simulink model "gm_parallel_lht_vnl"  (R2019b)
settings: Solver=FixedStepDiscrete  StartTime=0.0  StopTime=inf  RelTol=1e-3
undefined symbols (not defined in the file or in its folder): bt, height, nTheta, width
libraries: hdlsllib x199, simulink x27, hdlmdlgenlib x7, dspsrcs4 x1
(part 4 of 19)

== system gm_parallel_lht_vnl/Parallel LHT/Parallel LHT Accumulator/Accumulator with Switches/Accumulator_instance125 ==
  mode : Inport  OutDataTypeStr=boolean  PortDimensions=1  SampleTime=6.66666666666667e-09
  address : Inport  Port=2  OutDataTypeStr=fixdt(0, 9, 0)  PortDimensions=1  SampleTime=6.66666666666667e-09
  edge : Inport  Port=3  OutDataTypeStr=boolean  PortDimensions=1  SampleTime=6.66666666666667e-09
  AND : Logic  IconShape=distinctive  AllPortsSameDT=off  OutDataTypeStr=boolean
  Add : Sum  OutDataTypeStr=fixdt(0, ceil(log2(maxRho*2)), 0)
  Block RAM : Subsystem
  Delay{,1..3} (4 alike) : Delay  DelayLength=1
  Multiport Switch : MultiPortSwitch  DataPortOrder=Zero-based contiguous  Inputs=2  zeroidx=on
  Multiport Switch1 : MultiPortSwitch  DataPortOrder=Zero-based contiguous  Inputs=2  zeroidx=on
  Relational Operator : RelationalOperator  Operator===  OutDataTypeStr=boolean  RndMeth=Simplest
  Vote : Constant  OutDataTypeStr=fixdt(0,1,0)  SampleTime=-1
  Zero : Constant  OutDataTypeStr=fixdt(0,1,0)  SampleTime=-1
  hps : Outport
  wires:
  Zero/1 -> Multiport Switch/2
  Vote/1 -> Add/1
  Relational Operator/1 -> AND/2
  Delay2/1 -> Multiport Switch1/1
  Delay1/1 -> AND/1, Block RAM/3(wr_en)
  Delay/1 -> Relational Operator/1, Block RAM/2(wr_addr)
  Block RAM/1(rd_data) -> hps/1, Multiport Switch1/2
  AND/1 -> Delay2/1
  mode/1 -> Multiport Switch/1
  address/1 -> Relational Operator/2, Delay/1, Block RAM/4(rd_addr)
  edge/1 -> Delay1/1
  Multiport Switch/1 -> Block RAM/1(wr_data)
  Delay3/1 -> Multiport Switch1/3
  Multiport Switch1/1 -> Add/2
  Add/1 -> Multiport Switch/3, Delay3/1

== system gm_parallel_lht_vnl/Parallel LHT/Parallel LHT Accumulator/Accumulator with Switches/Accumulator_instance126 ==
  mode : Inport  OutDataTypeStr=boolean  PortDimensions=1  SampleTime=6.66666666666667e-09
  address : Inport  Port=2  OutDataTypeStr=fixdt(0, 9, 0)  PortDimensions=1  SampleTime=6.66666666666667e-09
  edge : Inport  Port=3  OutDataTypeStr=boolean  PortDimensions=1  SampleTime=6.66666666666667e-09
  AND : Logic  IconShape=distinctive  AllPortsSameDT=off  OutDataTypeStr=boolean
  Add : Sum  OutDataTypeStr=fixdt(0, ceil(log2(maxRho*2)), 0)
  Block RAM : Subsystem
  Delay{,1..3} (4 alike) : Delay  DelayLength=1
  Multiport Switch : MultiPortSwitch  DataPortOrder=Zero-based contiguous  Inputs=2  zeroidx=on
  Multiport Switch1 : MultiPortSwitch  DataPortOrder=Zero-based contiguous  Inputs=2  zeroidx=on
  Relational Operator : RelationalOperator  Operator===  OutDataTypeStr=boolean  RndMeth=Simplest
  Vote : Constant  OutDataTypeStr=fixdt(0,1,0)  SampleTime=-1
  Zero : Constant  OutDataTypeStr=fixdt(0,1,0)  SampleTime=-1
  hps : Outport
  wires:
  Zero/1 -> Multiport Switch/2
  Vote/1 -> Add/1
  Relational Operator/1 -> AND/2
  Delay2/1 -> Multiport Switch1/1
  Delay1/1 -> AND/1, Block RAM/3(wr_en)
  Delay/1 -> Relational Operator/1, Block RAM/2(wr_addr)
  Block RAM/1(rd_data) -> hps/1, Multiport Switch1/2
  AND/1 -> Delay2/1
  mode/1 -> Multiport Switch/1
  address/1 -> Relational Operator/2, Delay/1, Block RAM/4(rd_addr)
  edge/1 -> Delay1/1
  Multiport Switch/1 -> Block RAM/1(wr_data)
  Delay3/1 -> Multiport Switch1/3
  Multiport Switch1/1 -> Add/2
  Add/1 -> Multiport Switch/3, Delay3/1

== system gm_parallel_lht_vnl/Parallel LHT/Parallel LHT Accumulator/Accumulator with Switches/Accumulator_instance127 ==
  mode : Inport  OutDataTypeStr=boolean  PortDimensions=1  SampleTime=6.66666666666667e-09
  address : Inport  Port=2  OutDataTypeStr=fixdt(0, 9, 0)  PortDimensions=1  SampleTime=6.66666666666667e-09
  edge : Inport  Port=3  OutDataTypeStr=boolean  PortDimensions=1  SampleTime=6.66666666666667e-09
  AND : Logic  IconShape=distinctive  AllPortsSameDT=off  OutDataTypeStr=boolean
  Add : Sum  OutDataTypeStr=fixdt(0, ceil(log2(maxRho*2)), 0)
  Block RAM : Subsystem
  Delay{,1..3} (4 alike) : Delay  DelayLength=1
  Multiport Switch : MultiPortSwitch  DataPortOrder=Zero-based contiguous  Inputs=2  zeroidx=on
  Multiport Switch1 : MultiPortSwitch  DataPortOrder=Zero-based contiguous  Inputs=2  zeroidx=on
  Relational Operator : RelationalOperator  Operator===  OutDataTypeStr=boolean  RndMeth=Simplest
  Vote : Constant  OutDataTypeStr=fixdt(0,1,0)  SampleTime=-1
  Zero : Constant  OutDataTypeStr=fixdt(0,1,0)  SampleTime=-1
  hps : Outport
  wires:
  Zero/1 -> Multiport Switch/2
  Vote/1 -> Add/1
  Relational Operator/1 -> AND/2
  Delay2/1 -> Multiport Switch1/1
  Delay1/1 -> AND/1, Block RAM/3(wr_en)
  Delay/1 -> Relational Operator/1, Block RAM/2(wr_addr)
  Block RAM/1(rd_data) -> hps/1, Multiport Switch1/2
  AND/1 -> Delay2/1
  mode/1 -> Multiport Switch/1
  address/1 -> Relational Operator/2, Delay/1, Block RAM/4(rd_addr)
  edge/1 -> Delay1/1
  Multiport Switch/1 -> Block RAM/1(wr_data)
  Delay3/1 -> Multiport Switch1/3
  Multiport Switch1/1 -> Add/2
  Add/1 -> Multiport Switch/3, Delay3/1

== system gm_parallel_lht_vnl/Parallel LHT/Parallel LHT Accumulator/Accumulator with Switches/Accumulator_instance128 ==
  mode : Inport  OutDataTypeStr=boolean  PortDimensions=1  SampleTime=6.66666666666667e-09
  address : Inport  Port=2  OutDataTypeStr=fixdt(0, 9, 0)  PortDimensions=1  SampleTime=6.66666666666667e-09
  edge : Inport  Port=3  OutDataTypeStr=boolean  PortDimensions=1  SampleTime=6.66666666666667e-09
  AND : Logic  IconShape=distinctive  AllPortsSameDT=off  OutDataTypeStr=boolean
  Add : Sum  OutDataTypeStr=fixdt(0, ceil(log2(maxRho*2)), 0)
  Block RAM : Subsystem
  Delay{,1..3} (4 alike) : Delay  DelayLength=1
  Multiport Switch : MultiPortSwitch  DataPortOrder=Zero-based contiguous  Inputs=2  zeroidx=on
  Multiport Switch1 : MultiPortSwitch  DataPortOrder=Zero-based contiguous  Inputs=2  zeroidx=on
  Relational Operator : RelationalOperator  Operator===  OutDataTypeStr=boolean  RndMeth=Simplest
  Vote : Constant  OutDataTypeStr=fixdt(0,1,0)  SampleTime=-1
  Zero : Constant  OutDataTypeStr=fixdt(0,1,0)  SampleTime=-1
  hps : Outport
  wires:
  Zero/1 -> Multiport Switch/2
  Vote/1 -> Add/1
  Relational Operator/1 -> AND/2
  Delay2/1 -> Multiport Switch1/1
  Delay1/1 -> AND/1, Block RAM/3(wr_en)
  Delay/1 -> Relational Operator/1, Block RAM/2(wr_addr)
  Block RAM/1(rd_data) -> hps/1, Multiport Switch1/2
  AND/1 -> Delay2/1
  mode/1 -> Multiport Switch/1
  address/1 -> Relational Operator/2, Delay/1, Block RAM/4(rd_addr)
  edge/1 -> Delay1/1
  Multiport Switch/1 -> Block RAM/1(wr_data)
  Delay3/1 -> Multiport Switch1/3
  Multiport Switch1/1 -> Add/2
  Add/1 -> Multiport Switch/3, Delay3/1

== system gm_parallel_lht_vnl/Parallel LHT/Parallel LHT Accumulator/Accumulator with Switches/Accumulator_instance129 ==
  mode : Inport  OutDataTypeStr=boolean  PortDimensions=1  SampleTime=6.66666666666667e-09
  address : Inport  Port=2  OutDataTypeStr=fixdt(0, 9, 0)  PortDimensions=1  SampleTime=6.66666666666667e-09
  edge : Inport  Port=3  OutDataTypeStr=boolean  PortDimensions=1  SampleTime=6.66666666666667e-09
  AND : Logic  IconShape=distinctive  AllPortsSameDT=off  OutDataTypeStr=boolean
  Add : Sum  OutDataTypeStr=fixdt(0, ceil(log2(maxRho*2)), 0)
  Block RAM : Subsystem
  Delay{,1..3} (4 alike) : Delay  DelayLength=1
  Multiport Switch : MultiPortSwitch  DataPortOrder=Zero-based contiguous  Inputs=2  zeroidx=on
  Multiport Switch1 : MultiPortSwitch  DataPortOrder=Zero-based contiguous  Inputs=2  zeroidx=on
  Relational Operator : RelationalOperator  Operator===  OutDataTypeStr=boolean  RndMeth=Simplest
  Vote : Constant  OutDataTypeStr=fixdt(0,1,0)  SampleTime=-1
  Zero : Constant  OutDataTypeStr=fixdt(0,1,0)  SampleTime=-1
  hps : Outport
  wires:
  Zero/1 -> Multiport Switch/2
  Vote/1 -> Add/1
  Relational Operator/1 -> AND/2
  Delay2/1 -> Multiport Switch1/1
  Delay1/1 -> AND/1, Block RAM/3(wr_en)
  Delay/1 -> Relational Operator/1, Block RAM/2(wr_addr)
  Block RAM/1(rd_data) -> hps/1, Multiport Switch1/2
  AND/1 -> Delay2/1
  mode/1 -> Multiport Switch/1
  address/1 -> Relational Operator/2, Delay/1, Block RAM/4(rd_addr)
  edge/1 -> Delay1/1
  Multiport Switch/1 -> Block RAM/1(wr_data)
  Delay3/1 -> Multiport Switch1/3
  Multiport Switch1/1 -> Add/2
  Add/1 -> Multiport Switch/3, Delay3/1

== system gm_parallel_lht_vnl/Parallel LHT/Parallel LHT Accumulator/Accumulator with Switches/Accumulator_instance13 ==
  mode : Inport  OutDataTypeStr=boolean  PortDimensions=1  SampleTime=6.66666666666667e-09
  address : Inport  Port=2  OutDataTypeStr=fixdt(0, 9, 0)  PortDimensions=1  SampleTime=6.66666666666667e-09
  edge : Inport  Port=3  OutDataTypeStr=boolean  PortDimensions=1  SampleTime=6.66666666666667e-09
  AND : Logic  IconShape=distinctive  AllPortsSameDT=off  OutDataTypeStr=boolean
  Add : Sum  OutDataTypeStr=fixdt(0, ceil(log2(maxRho*2)), 0)
  Block RAM : Subsystem
  Delay{,1..3} (4 alike) : Delay  DelayLength=1
  Multiport Switch : MultiPortSwitch  DataPortOrder=Zero-based contiguous  Inputs=2  zeroidx=on
  Multiport Switch1 : MultiPortSwitch  DataPortOrder=Zero-based contiguous  Inputs=2  zeroidx=on
  Relational Operator : RelationalOperator  Operator===  OutDataTypeStr=boolean  RndMeth=Simplest
  Vote : Constant  OutDataTypeStr=fixdt(0,1,0)  SampleTime=-1
  Zero : Constant  OutDataTypeStr=fixdt(0,1,0)  SampleTime=-1
  hps : Outport
  wires:
  Zero/1 -> Multiport Switch/2
  Vote/1 -> Add/1
  Relational Operator/1 -> AND/2
  Delay2/1 -> Multiport Switch1/1
  Delay1/1 -> AND/1, Block RAM/3(wr_en)
  Delay/1 -> Relational Operator/1, Block RAM/2(wr_addr)
  Block RAM/1(rd_data) -> hps/1, Multiport Switch1/2
  AND/1 -> Delay2/1
  mode/1 -> Multiport Switch/1
  address/1 -> Relational Operator/2, Delay/1, Block RAM/4(rd_addr)
  edge/1 -> Delay1/1
  Multiport Switch/1 -> Block RAM/1(wr_data)
  Delay3/1 -> Multiport Switch1/3
  Multiport Switch1/1 -> Add/2
  Add/1 -> Multiport Switch/3, Delay3/1

== system gm_parallel_lht_vnl/Parallel LHT/Parallel LHT Accumulator/Accumulator with Switches/Accumulator_instance130 ==
  mode : Inport  OutDataTypeStr=boolean  PortDimensions=1  SampleTime=6.66666666666667e-09
  address : Inport  Port=2  OutDataTypeStr=fixdt(0, 9, 0)  PortDimensions=1  SampleTime=6.66666666666667e-09
  edge : Inport  Port=3  OutDataTypeStr=boolean  PortDimensions=1  SampleTime=6.66666666666667e-09
  AND : Logic  IconShape=distinctive  AllPortsSameDT=off  OutDataTypeStr=boolean
  Add : Sum  OutDataTypeStr=fixdt(0, ceil(log2(maxRho*2)), 0)
  Block RAM : Subsystem
  Delay{,1..3} (4 alike) : Delay  DelayLength=1
  Multiport Switch : MultiPortSwitch  DataPortOrder=Zero-based contiguous  Inputs=2  zeroidx=on
  Multiport Switch1 : MultiPortSwitch  DataPortOrder=Zero-based contiguous  Inputs=2  zeroidx=on
  Relational Operator : RelationalOperator  Operator===  OutDataTypeStr=boolean  RndMeth=Simplest
  Vote : Constant  OutDataTypeStr=fixdt(0,1,0)  SampleTime=-1
  Zero : Constant  OutDataTypeStr=fixdt(0,1,0)  SampleTime=-1
  hps : Outport
  wires:
  Zero/1 -> Multiport Switch/2
  Vote/1 -> Add/1
  Relational Operator/1 -> AND/2
  Delay2/1 -> Multiport Switch1/1
  Delay1/1 -> AND/1, Block RAM/3(wr_en)
  Delay/1 -> Relational Operator/1, Block RAM/2(wr_addr)
  Block RAM/1(rd_data) -> hps/1, Multiport Switch1/2
  AND/1 -> Delay2/1
  mode/1 -> Multiport Switch/1
  address/1 -> Relational Operator/2, Delay/1, Block RAM/4(rd_addr)
  edge/1 -> Delay1/1
  Multiport Switch/1 -> Block RAM/1(wr_data)
  Delay3/1 -> Multiport Switch1/3
  Multiport Switch1/1 -> Add/2
  Add/1 -> Multiport Switch/3, Delay3/1

== system gm_parallel_lht_vnl/Parallel LHT/Parallel LHT Accumulator/Accumulator with Switches/Accumulator_instance131 ==
  mode : Inport  OutDataTypeStr=boolean  PortDimensions=1  SampleTime=6.66666666666667e-09
  address : Inport  Port=2  OutDataTypeStr=fixdt(0, 9, 0)  PortDimensions=1  SampleTime=6.66666666666667e-09
  edge : Inport  Port=3  OutDataTypeStr=boolean  PortDimensions=1  SampleTime=6.66666666666667e-09
  AND : Logic  IconShape=distinctive  AllPortsSameDT=off  OutDataTypeStr=boolean
  Add : Sum  OutDataTypeStr=fixdt(0, ceil(log2(maxRho*2)), 0)
  Block RAM : Subsystem
  Delay{,1..3} (4 alike) : Delay  DelayLength=1
  Multiport Switch : MultiPortSwitch  DataPortOrder=Zero-based contiguous  Inputs=2  zeroidx=on
  Multiport Switch1 : MultiPortSwitch  DataPortOrder=Zero-based contiguous  Inputs=2  zeroidx=on
  Relational Operator : RelationalOperator  Operator===  OutDataTypeStr=boolean  RndMeth=Simplest
  Vote : Constant  OutDataTypeStr=fixdt(0,1,0)  SampleTime=-1
  Zero : Constant  OutDataTypeStr=fixdt(0,1,0)  SampleTime=-1
  hps : Outport
  wires:
  Zero/1 -> Multiport Switch/2
  Vote/1 -> Add/1
  Relational Operator/1 -> AND/2
  Delay2/1 -> Multiport Switch1/1
  Delay1/1 -> AND/1, Block RAM/3(wr_en)
  Delay/1 -> Relational Operator/1, Block RAM/2(wr_addr)
  Block RAM/1(rd_data) -> hps/1, Multiport Switch1/2
  AND/1 -> Delay2/1
  mode/1 -> Multiport Switch/1
  address/1 -> Relational Operator/2, Delay/1, Block RAM/4(rd_addr)
  edge/1 -> Delay1/1
  Multiport Switch/1 -> Block RAM/1(wr_data)
  Delay3/1 -> Multiport Switch1/3
  Multiport Switch1/1 -> Add/2
  Add/1 -> Multiport Switch/3, Delay3/1

== system gm_parallel_lht_vnl/Parallel LHT/Parallel LHT Accumulator/Accumulator with Switches/Accumulator_instance132 ==
  mode : Inport  OutDataTypeStr=boolean  PortDimensions=1  SampleTime=6.66666666666667e-09
  address : Inport  Port=2  OutDataTypeStr=fixdt(0, 9, 0)  PortDimensions=1  SampleTime=6.66666666666667e-09
  edge : Inport  Port=3  OutDataTypeStr=boolean  PortDimensions=1  SampleTime=6.66666666666667e-09
  AND : Logic  IconShape=distinctive  AllPortsSameDT=off  OutDataTypeStr=boolean
  Add : Sum  OutDataTypeStr=fixdt(0, ceil(log2(maxRho*2)), 0)
  Block RAM : Subsystem
  Delay{,1..3} (4 alike) : Delay  DelayLength=1
  Multiport Switch : MultiPortSwitch  DataPortOrder=Zero-based contiguous  Inputs=2  zeroidx=on
  Multiport Switch1 : MultiPortSwitch  DataPortOrder=Zero-based contiguous  Inputs=2  zeroidx=on
  Relational Operator : RelationalOperator  Operator===  OutDataTypeStr=boolean  RndMeth=Simplest
  Vote : Constant  OutDataTypeStr=fixdt(0,1,0)  SampleTime=-1
  Zero : Constant  OutDataTypeStr=fixdt(0,1,0)  SampleTime=-1
  hps : Outport
  wires:
  Zero/1 -> Multiport Switch/2
  Vote/1 -> Add/1
  Relational Operator/1 -> AND/2
  Delay2/1 -> Multiport Switch1/1
  Delay1/1 -> AND/1, Block RAM/3(wr_en)
  Delay/1 -> Relational Operator/1, Block RAM/2(wr_addr)
  Block RAM/1(rd_data) -> hps/1, Multiport Switch1/2
  AND/1 -> Delay2/1
  mode/1 -> Multiport Switch/1
  address/1 -> Relational Operator/2, Delay/1, Block RAM/4(rd_addr)
  edge/1 -> Delay1/1
  Multiport Switch/1 -> Block RAM/1(wr_data)
  Delay3/1 -> Multiport Switch1/3
  Multiport Switch1/1 -> Add/2
  Add/1 -> Multiport Switch/3, Delay3/1

== system gm_parallel_lht_vnl/Parallel LHT/Parallel LHT Accumulator/Accumulator with Switches/Accumulator_instance133 ==
  mode : Inport  OutDataTypeStr=boolean  PortDimensions=1  SampleTime=6.66666666666667e-09
  address : Inport  Port=2  OutDataTypeStr=fixdt(0, 9, 0)  PortDimensions=1  SampleTime=6.66666666666667e-09
  edge : Inport  Port=3  OutDataTypeStr=boolean  PortDimensions=1  SampleTime=6.66666666666667e-09
  AND : Logic  IconShape=distinctive  AllPortsSameDT=off  OutDataTypeStr=boolean
  Add : Sum  OutDataTypeStr=fixdt(0, ceil(log2(maxRho*2)), 0)
  Block RAM : Subsystem
  Delay{,1..3} (4 alike) : Delay  DelayLength=1
  Multiport Switch : MultiPortSwitch  DataPortOrder=Zero-based contiguous  Inputs=2  zeroidx=on
  Multiport Switch1 : MultiPortSwitch  DataPortOrder=Zero-based contiguous  Inputs=2  zeroidx=on
  Relational Operator : RelationalOperator  Operator===  OutDataTypeStr=boolean  RndMeth=Simplest
  Vote : Constant  OutDataTypeStr=fixdt(0,1,0)  SampleTime=-1
  Zero : Constant  OutDataTypeStr=fixdt(0,1,0)  SampleTime=-1
  hps : Outport
  wires:
  Zero/1 -> Multiport Switch/2
  Vote/1 -> Add/1
  Relational Operator/1 -> AND/2
  Delay2/1 -> Multiport Switch1/1
  Delay1/1 -> AND/1, Block RAM/3(wr_en)
  Delay/1 -> Relational Operator/1, Block RAM/2(wr_addr)
  Block RAM/1(rd_data) -> hps/1, Multiport Switch1/2
  AND/1 -> Delay2/1
  mode/1 -> Multiport Switch/1
  address/1 -> Relational Operator/2, Delay/1, Block RAM/4(rd_addr)
  edge/1 -> Delay1/1
  Multiport Switch/1 -> Block RAM/1(wr_data)
  Delay3/1 -> Multiport Switch1/3
  Multiport Switch1/1 -> Add/2
  Add/1 -> Multiport Switch/3, Delay3/1

== system gm_parallel_lht_vnl/Parallel LHT/Parallel LHT Accumulator/Accumulator with Switches/Accumulator_instance134 ==
  mode : Inport  OutDataTypeStr=boolean  PortDimensions=1  SampleTime=6.66666666666667e-09
  address : Inport  Port=2  OutDataTypeStr=fixdt(0, 9, 0)  PortDimensions=1  SampleTime=6.66666666666667e-09
  edge : Inport  Port=3  OutDataTypeStr=boolean  PortDimensions=1  SampleTime=6.66666666666667e-09
  AND : Logic  IconShape=distinctive  AllPortsSameDT=off  OutDataTypeStr=boolean
  Add : Sum  OutDataTypeStr=fixdt(0, ceil(log2(maxRho*2)), 0)
  Block RAM : Subsystem
  Delay{,1..3} (4 alike) : Delay  DelayLength=1
  Multiport Switch : MultiPortSwitch  DataPortOrder=Zero-based contiguous  Inputs=2  zeroidx=on
  Multiport Switch1 : MultiPortSwitch  DataPortOrder=Zero-based contiguous  Inputs=2  zeroidx=on
  Relational Operator : RelationalOperator  Operator===  OutDataTypeStr=boolean  RndMeth=Simplest
  Vote : Constant  OutDataTypeStr=fixdt(0,1,0)  SampleTime=-1
  Zero : Constant  OutDataTypeStr=fixdt(0,1,0)  SampleTime=-1
  hps : Outport
  wires:
  Zero/1 -> Multiport Switch/2
  Vote/1 -> Add/1
  Relational Operator/1 -> AND/2
  Delay2/1 -> Multiport Switch1/1
  Delay1/1 -> AND/1, Block RAM/3(wr_en)
  Delay/1 -> Relational Operator/1, Block RAM/2(wr_addr)
  Block RAM/1(rd_data) -> hps/1, Multiport Switch1/2
  AND/1 -> Delay2/1
  mode/1 -> Multiport Switch/1
  address/1 -> Relational Operator/2, Delay/1, Block RAM/4(rd_addr)
  edge/1 -> Delay1/1
  Multiport Switch/1 -> Block RAM/1(wr_data)
  Delay3/1 -> Multiport Switch1/3
  Multiport Switch1/1 -> Add/2
  Add/1 -> Multiport Switch/3, Delay3/1

== system gm_parallel_lht_vnl/Parallel LHT/Parallel LHT Accumulator/Accumulator with Switches/Accumulator_instance135 ==
  mode : Inport  OutDataTypeStr=boolean  PortDimensions=1  SampleTime=6.66666666666667e-09
  address : Inport  Port=2  OutDataTypeStr=fixdt(0, 9, 0)  PortDimensions=1  SampleTime=6.66666666666667e-09
  edge : Inport  Port=3  OutDataTypeStr=boolean  PortDimensions=1  SampleTime=6.66666666666667e-09
  AND : Logic  IconShape=distinctive  AllPortsSameDT=off  OutDataTypeStr=boolean
  Add : Sum  OutDataTypeStr=fixdt(0, ceil(log2(maxRho*2)), 0)
  Block RAM : Subsystem
  Delay{,1..3} (4 alike) : Delay  DelayLength=1
  Multiport Switch : MultiPortSwitch  DataPortOrder=Zero-based contiguous  Inputs=2  zeroidx=on
  Multiport Switch1 : MultiPortSwitch  DataPortOrder=Zero-based contiguous  Inputs=2  zeroidx=on
  Relational Operator : RelationalOperator  Operator===  OutDataTypeStr=boolean  RndMeth=Simplest
  Vote : Constant  OutDataTypeStr=fixdt(0,1,0)  SampleTime=-1
  Zero : Constant  OutDataTypeStr=fixdt(0,1,0)  SampleTime=-1
  hps : Outport
  wires:
  Zero/1 -> Multiport Switch/2
  Vote/1 -> Add/1
  Relational Operator/1 -> AND/2
  Delay2/1 -> Multiport Switch1/1
  Delay1/1 -> AND/1, Block RAM/3(wr_en)
  Delay/1 -> Relational Operator/1, Block RAM/2(wr_addr)
  Block RAM/1(rd_data) -> hps/1, Multiport Switch1/2
  AND/1 -> Delay2/1
  mode/1 -> Multiport Switch/1
  address/1 -> Relational Operator/2, Delay/1, Block RAM/4(rd_addr)
  edge/1 -> Delay1/1
  Multiport Switch/1 -> Block RAM/1(wr_data)
  Delay3/1 -> Multiport Switch1/3
  Multiport Switch1/1 -> Add/2
  Add/1 -> Multiport Switch/3, Delay3/1

== system gm_parallel_lht_vnl/Parallel LHT/Parallel LHT Accumulator/Accumulator with Switches/Accumulator_instance136 ==
  mode : Inport  OutDataTypeStr=boolean  PortDimensions=1  SampleTime=6.66666666666667e-09
  address : Inport  Port=2  OutDataTypeStr=fixdt(0, 9, 0)  PortDimensions=1  SampleTime=6.66666666666667e-09
  edge : Inport  Port=3  OutDataTypeStr=boolean  PortDimensions=1  SampleTime=6.66666666666667e-09
  AND : Logic  IconShape=distinctive  AllPortsSameDT=off  OutDataTypeStr=boolean
  Add : Sum  OutDataTypeStr=fixdt(0, ceil(log2(maxRho*2)), 0)
  Block RAM : Subsystem
  Delay{,1..3} (4 alike) : Delay  DelayLength=1
  Multiport Switch : MultiPortSwitch  DataPortOrder=Zero-based contiguous  Inputs=2  zeroidx=on
  Multiport Switch1 : MultiPortSwitch  DataPortOrder=Zero-based contiguous  Inputs=2  zeroidx=on
  Relational Operator : RelationalOperator  Operator===  OutDataTypeStr=boolean  RndMeth=Simplest
  Vote : Constant  OutDataTypeStr=fixdt(0,1,0)  SampleTime=-1
  Zero : Constant  OutDataTypeStr=fixdt(0,1,0)  SampleTime=-1
  hps : Outport
  wires:
  Zero/1 -> Multiport Switch/2
  Vote/1 -> Add/1
  Relational Operator/1 -> AND/2
  Delay2/1 -> Multiport Switch1/1
  Delay1/1 -> AND/1, Block RAM/3(wr_en)
  Delay/1 -> Relational Operator/1, Block RAM/2(wr_addr)
  Block RAM/1(rd_data) -> hps/1, Multiport Switch1/2
  AND/1 -> Delay2/1
  mode/1 -> Multiport Switch/1
  address/1 -> Relational Operator/2, Delay/1, Block RAM/4(rd_addr)
  edge/1 -> Delay1/1
  Multiport Switch/1 -> Block RAM/1(wr_data)
  Delay3/1 -> Multiport Switch1/3
  Multiport Switch1/1 -> Add/2
  Add/1 -> Multiport Switch/3, Delay3/1

== system gm_parallel_lht_vnl/Parallel LHT/Parallel LHT Accumulator/Accumulator with Switches/Accumulator_instance137 ==
  mode : Inport  OutDataTypeStr=boolean  PortDimensions=1  SampleTime=6.66666666666667e-09
  address : Inport  Port=2  OutDataTypeStr=fixdt(0, 9, 0)  PortDimensions=1  SampleTime=6.66666666666667e-09
  edge : Inport  Port=3  OutDataTypeStr=boolean  PortDimensions=1  SampleTime=6.66666666666667e-09
  AND : Logic  IconShape=distinctive  AllPortsSameDT=off  OutDataTypeStr=boolean
  Add : Sum  OutDataTypeStr=fixdt(0, ceil(log2(maxRho*2)), 0)
  Block RAM : Subsystem
  Delay{,1..3} (4 alike) : Delay  DelayLength=1
  Multiport Switch : MultiPortSwitch  DataPortOrder=Zero-based contiguous  Inputs=2  zeroidx=on
  Multiport Switch1 : MultiPortSwitch  DataPortOrder=Zero-based contiguous  Inputs=2  zeroidx=on
  Relational Operator : RelationalOperator  Operator===  OutDataTypeStr=boolean  RndMeth=Simplest
  Vote : Constant  OutDataTypeStr=fixdt(0,1,0)  SampleTime=-1
  Zero : Constant  OutDataTypeStr=fixdt(0,1,0)  SampleTime=-1
  hps : Outport
  wires:
  Zero/1 -> Multiport Switch/2
  Vote/1 -> Add/1
  Relational Operator/1 -> AND/2
  Delay2/1 -> Multiport Switch1/1
  Delay1/1 -> AND/1, Block RAM/3(wr_en)
  Delay/1 -> Relational Operator/1, Block RAM/2(wr_addr)
  Block RAM/1(rd_data) -> hps/1, Multiport Switch1/2
  AND/1 -> Delay2/1
  mode/1 -> Multiport Switch/1
  address/1 -> Relational Operator/2, Delay/1, Block RAM/4(rd_addr)
  edge/1 -> Delay1/1
  Multiport Switch/1 -> Block RAM/1(wr_data)
  Delay3/1 -> Multiport Switch1/3
  Multiport Switch1/1 -> Add/2
  Add/1 -> Multiport Switch/3, Delay3/1

== system gm_parallel_lht_vnl/Parallel LHT/Parallel LHT Accumulator/Accumulator with Switches/Accumulator_instance138 ==
  mode : Inport  OutDataTypeStr=boolean  PortDimensions=1  SampleTime=6.66666666666667e-09
  address : Inport  Port=2  OutDataTypeStr=fixdt(0, 9, 0)  PortDimensions=1  SampleTime=6.66666666666667e-09
  edge : Inport  Port=3  OutDataTypeStr=boolean  PortDimensions=1  SampleTime=6.66666666666667e-09
  AND : Logic  IconShape=distinctive  AllPortsSameDT=off  OutDataTypeStr=boolean
  Add : Sum  OutDataTypeStr=fixdt(0, ceil(log2(maxRho*2)), 0)
  Block RAM : Subsystem
  Delay{,1..3} (4 alike) : Delay  DelayLength=1
  Multiport Switch : MultiPortSwitch  DataPortOrder=Zero-based contiguous  Inputs=2  zeroidx=on
  Multiport Switch1 : MultiPortSwitch  DataPortOrder=Zero-based contiguous  Inputs=2  zeroidx=on
  Relational Operator : RelationalOperator  Operator===  OutDataTypeStr=boolean  RndMeth=Simplest
  Vote : Constant  OutDataTypeStr=fixdt(0,1,0)  SampleTime=-1
  Zero : Constant  OutDataTypeStr=fixdt(0,1,0)  SampleTime=-1
  hps : Outport
  wires:
  Zero/1 -> Multiport Switch/2
  Vote/1 -> Add/1
  Relational Operator/1 -> AND/2
  Delay2/1 -> Multiport Switch1/1
  Delay1/1 -> AND/1, Block RAM/3(wr_en)
  Delay/1 -> Relational Operator/1, Block RAM/2(wr_addr)
  Block RAM/1(rd_data) -> hps/1, Multiport Switch1/2
  AND/1 -> Delay2/1
  mode/1 -> Multiport Switch/1
  address/1 -> Relational Operator/2, Delay/1, Block RAM/4(rd_addr)
  edge/1 -> Delay1/1
  Multiport Switch/1 -> Block RAM/1(wr_data)
  Delay3/1 -> Multiport Switch1/3
  Multiport Switch1/1 -> Add/2
  Add/1 -> Multiport Switch/3, Delay3/1

== system gm_parallel_lht_vnl/Parallel LHT/Parallel LHT Accumulator/Accumulator with Switches/Accumulator_instance139 ==
  mode : Inport  OutDataTypeStr=boolean  PortDimensions=1  SampleTime=6.66666666666667e-09
  address : Inport  Port=2  OutDataTypeStr=fixdt(0, 9, 0)  PortDimensions=1  SampleTime=6.66666666666667e-09
  edge : Inport  Port=3  OutDataTypeStr=boolean  PortDimensions=1  SampleTime=6.66666666666667e-09
  AND : Logic  IconShape=distinctive  AllPortsSameDT=off  OutDataTypeStr=boolean
  Add : Sum  OutDataTypeStr=fixdt(0, ceil(log2(maxRho*2)), 0)
  Block RAM : Subsystem
  Delay{,1..3} (4 alike) : Delay  DelayLength=1
  Multiport Switch : MultiPortSwitch  DataPortOrder=Zero-based contiguous  Inputs=2  zeroidx=on
  Multiport Switch1 : MultiPortSwitch  DataPortOrder=Zero-based contiguous  Inputs=2  zeroidx=on
  Relational Operator : RelationalOperator  Operator===  OutDataTypeStr=boolean  RndMeth=Simplest
  Vote : Constant  OutDataTypeStr=fixdt(0,1,0)  SampleTime=-1
  Zero : Constant  OutDataTypeStr=fixdt(0,1,0)  SampleTime=-1
  hps : Outport
  wires:
  Zero/1 -> Multiport Switch/2
  Vote/1 -> Add/1
  Relational Operator/1 -> AND/2
  Delay2/1 -> Multiport Switch1/1
  Delay1/1 -> AND/1, Block RAM/3(wr_en)
  Delay/1 -> Relational Operator/1, Block RAM/2(wr_addr)
  Block RAM/1(rd_data) -> hps/1, Multiport Switch1/2
  AND/1 -> Delay2/1
  mode/1 -> Multiport Switch/1
  address/1 -> Relational Operator/2, Delay/1, Block RAM/4(rd_addr)
  edge/1 -> Delay1/1
  Multiport Switch/1 -> Block RAM/1(wr_data)
  Delay3/1 -> Multiport Switch1/3
  Multiport Switch1/1 -> Add/2
  Add/1 -> Multiport Switch/3, Delay3/1

== system gm_parallel_lht_vnl/Parallel LHT/Parallel LHT Accumulator/Accumulator with Switches/Accumulator_instance14 ==
  mode : Inport  OutDataTypeStr=boolean  PortDimensions=1  SampleTime=6.66666666666667e-09
  address : Inport  Port=2  OutDataTypeStr=fixdt(0, 9, 0)  PortDimensions=1  SampleTime=6.66666666666667e-09
  edge : Inport  Port=3  OutDataTypeStr=boolean  PortDimensions=1  SampleTime=6.66666666666667e-09
  AND : Logic  IconShape=distinctive  AllPortsSameDT=off  OutDataTypeStr=boolean
  Add : Sum  OutDataTypeStr=fixdt(0, ceil(log2(maxRho*2)), 0)
  Block RAM : Subsystem
  Delay{,1..3} (4 alike) : Delay  DelayLength=1
  Multiport Switch : MultiPortSwitch  DataPortOrder=Zero-based contiguous  Inputs=2  zeroidx=on
  Multiport Switch1 : MultiPortSwitch  DataPortOrder=Zero-based contiguous  Inputs=2  zeroidx=on
  Relational Operator : RelationalOperator  Operator===  OutDataTypeStr=boolean  RndMeth=Simplest
  Vote : Constant  OutDataTypeStr=fixdt(0,1,0)  SampleTime=-1
  Zero : Constant  OutDataTypeStr=fixdt(0,1,0)  SampleTime=-1
  hps : Outport
  wires:
  Zero/1 -> Multiport Switch/2
  Vote/1 -> Add/1
  Relational Operator/1 -> AND/2
  Delay2/1 -> Multiport Switch1/1
  Delay1/1 -> AND/1, Block RAM/3(wr_en)
  Delay/1 -> Relational Operator/1, Block RAM/2(wr_addr)
  Block RAM/1(rd_data) -> hps/1, Multiport Switch1/2
  AND/1 -> Delay2/1
  mode/1 -> Multiport Switch/1
  address/1 -> Relational Operator/2, Delay/1, Block RAM/4(rd_addr)
  edge/1 -> Delay1/1
  Multiport Switch/1 -> Block RAM/1(wr_data)
  Delay3/1 -> Multiport Switch1/3
  Multiport Switch1/1 -> Add/2
  Add/1 -> Multiport Switch/3, Delay3/1

== system gm_parallel_lht_vnl/Parallel LHT/Parallel LHT Accumulator/Accumulator with Switches/Accumulator_instance140 ==
  mode : Inport  OutDataTypeStr=boolean  PortDimensions=1  SampleTime=6.66666666666667e-09
  address : Inport  Port=2  OutDataTypeStr=fixdt(0, 9, 0)  PortDimensions=1  SampleTime=6.66666666666667e-09
  edge : Inport  Port=3  OutDataTypeStr=boolean  PortDimensions=1  SampleTime=6.66666666666667e-09
  AND : Logic  IconShape=distinctive  AllPortsSameDT=off  OutDataTypeStr=boolean
  Add : Sum  OutDataTypeStr=fixdt(0, ceil(log2(maxRho*2)), 0)
  Block RAM : Subsystem
  Delay{,1..3} (4 alike) : Delay  DelayLength=1
  Multiport Switch : MultiPortSwitch  DataPortOrder=Zero-based contiguous  Inputs=2  zeroidx=on
  Multiport Switch1 : MultiPortSwitch  DataPortOrder=Zero-based contiguous  Inputs=2  zeroidx=on
  Relational Operator : RelationalOperator  Operator===  OutDataTypeStr=boolean  RndMeth=Simplest
  Vote : Constant  OutDataTypeStr=fixdt(0,1,0)  SampleTime=-1
  Zero : Constant  OutDataTypeStr=fixdt(0,1,0)  SampleTime=-1
  hps : Outport
  wires:
  Zero/1 -> Multiport Switch/2
  Vote/1 -> Add/1
  Relational Operator/1 -> AND/2
  Delay2/1 -> Multiport Switch1/1
  Delay1/1 -> AND/1, Block RAM/3(wr_en)
  Delay/1 -> Relational Operator/1, Block RAM/2(wr_addr)
  Block RAM/1(rd_data) -> hps/1, Multiport Switch1/2
  AND/1 -> Delay2/1
  mode/1 -> Multiport Switch/1
  address/1 -> Relational Operator/2, Delay/1, Block RAM/4(rd_addr)
  edge/1 -> Delay1/1
  Multiport Switch/1 -> Block RAM/1(wr_data)
  Delay3/1 -> Multiport Switch1/3
  Multiport Switch1/1 -> Add/2
  Add/1 -> Multiport Switch/3, Delay3/1

== system gm_parallel_lht_vnl/Parallel LHT/Parallel LHT Accumulator/Accumulator with Switches/Accumulator_instance141 ==
  mode : Inport  OutDataTypeStr=boolean  PortDimensions=1  SampleTime=6.66666666666667e-09
  address : Inport  Port=2  OutDataTypeStr=fixdt(0, 9, 0)  PortDimensions=1  SampleTime=6.66666666666667e-09
  edge : Inport  Port=3  OutDataTypeStr=boolean  PortDimensions=1  SampleTime=6.66666666666667e-09
  AND : Logic  IconShape=distinctive  AllPortsSameDT=off  OutDataTypeStr=boolean
  Add : Sum  OutDataTypeStr=fixdt(0, ceil(log2(maxRho*2)), 0)
  Block RAM : Subsystem
  Delay{,1..3} (4 alike) : Delay  DelayLength=1
  Multiport Switch : MultiPortSwitch  DataPortOrder=Zero-based contiguous  Inputs=2  zeroidx=on
  Multiport Switch1 : MultiPortSwitch  DataPortOrder=Zero-based contiguous  Inputs=2  zeroidx=on
  Relational Operator : RelationalOperator  Operator===  OutDataTypeStr=boolean  RndMeth=Simplest
  Vote : Constant  OutDataTypeStr=fixdt(0,1,0)  SampleTime=-1
  Zero : Constant  OutDataTypeStr=fixdt(0,1,0)  SampleTime=-1
  hps : Outport
  wires:
  Zero/1 -> Multiport Switch/2
  Vote/1 -> Add/1
  Relational Operator/1 -> AND/2
  Delay2/1 -> Multiport Switch1/1
  Delay1/1 -> AND/1, Block RAM/3(wr_en)
  Delay/1 -> Relational Operator/1, Block RAM/2(wr_addr)
  Block RAM/1(rd_data) -> hps/1, Multiport Switch1/2
  AND/1 -> Delay2/1
  mode/1 -> Multiport Switch/1
  address/1 -> Relational Operator/2, Delay/1, Block RAM/4(rd_addr)
  edge/1 -> Delay1/1
  Multiport Switch/1 -> Block RAM/1(wr_data)
  Delay3/1 -> Multiport Switch1/3
  Multiport Switch1/1 -> Add/2
  Add/1 -> Multiport Switch/3, Delay3/1

== system gm_parallel_lht_vnl/Parallel LHT/Parallel LHT Accumulator/Accumulator with Switches/Accumulator_instance142 ==
  mode : Inport  OutDataTypeStr=boolean  PortDimensions=1  SampleTime=6.66666666666667e-09
  address : Inport  Port=2  OutDataTypeStr=fixdt(0, 9, 0)  PortDimensions=1  SampleTime=6.66666666666667e-09
  edge : Inport  Port=3  OutDataTypeStr=boolean  PortDimensions=1  SampleTime=6.66666666666667e-09
  AND : Logic  IconShape=distinctive  AllPortsSameDT=off  OutDataTypeStr=boolean
  Add : Sum  OutDataTypeStr=fixdt(0, ceil(log2(maxRho*2)), 0)
  Block RAM : Subsystem
  Delay{,1..3} (4 alike) : Delay  DelayLength=1
  Multiport Switch : MultiPortSwitch  DataPortOrder=Zero-based contiguous  Inputs=2  zeroidx=on
  Multiport Switch1 : MultiPortSwitch  DataPortOrder=Zero-based contiguous  Inputs=2  zeroidx=on
  Relational Operator : RelationalOperator  Operator===  OutDataTypeStr=boolean  RndMeth=Simplest
  Vote : Constant  OutDataTypeStr=fixdt(0,1,0)  SampleTime=-1
  Zero : Constant  OutDataTypeStr=fixdt(0,1,0)  SampleTime=-1
  hps : Outport
  wires:
  Zero/1 -> Multiport Switch/2
  Vote/1 -> Add/1
  Relational Operator/1 -> AND/2
  Delay2/1 -> Multiport Switch1/1
  Delay1/1 -> AND/1, Block RAM/3(wr_en)
  Delay/1 -> Relational Operator/1, Block RAM/2(wr_addr)
  Block RAM/1(rd_data) -> hps/1, Multiport Switch1/2
  AND/1 -> Delay2/1
  mode/1 -> Multiport Switch/1
  address/1 -> Relational Operator/2, Delay/1, Block RAM/4(rd_addr)
  edge/1 -> Delay1/1
  Multiport Switch/1 -> Block RAM/1(wr_data)
  Delay3/1 -> Multiport Switch1/3
  Multiport Switch1/1 -> Add/2
  Add/1 -> Multiport Switch/3, Delay3/1

== system gm_parallel_lht_vnl/Parallel LHT/Parallel LHT Accumulator/Accumulator with Switches/Accumulator_instance143 ==
  mode : Inport  OutDataTypeStr=boolean  PortDimensions=1  SampleTime=6.66666666666667e-09
  address : Inport  Port=2  OutDataTypeStr=fixdt(0, 9, 0)  PortDimensions=1  SampleTime=6.66666666666667e-09
  edge : Inport  Port=3  OutDataTypeStr=boolean  PortDimensions=1  SampleTime=6.66666666666667e-09
  AND : Logic  IconShape=distinctive  AllPortsSameDT=off  OutDataTypeStr=boolean
  Add : Sum  OutDataTypeStr=fixdt(0, ceil(log2(maxRho*2)), 0)
  Block RAM : Subsystem
  Delay{,1..3} (4 alike) : Delay  DelayLength=1
  Multiport Switch : MultiPortSwitch  DataPortOrder=Zero-based contiguous  Inputs=2  zeroidx=on
  Multiport Switch1 : MultiPortSwitch  DataPortOrder=Zero-based contiguous  Inputs=2  zeroidx=on
  Relational Operator : RelationalOperator  Operator===  OutDataTypeStr=boolean  RndMeth=Simplest
  Vote : Constant  OutDataTypeStr=fixdt(0,1,0)  SampleTime=-1
  Zero : Constant  OutDataTypeStr=fixdt(0,1,0)  SampleTime=-1
  hps : Outport
  wires:
  Zero/1 -> Multiport Switch/2
  Vote/1 -> Add/1
  Relational Operator/1 -> AND/2
  Delay2/1 -> Multiport Switch1/1
  Delay1/1 -> AND/1, Block RAM/3(wr_en)
  Delay/1 -> Relational Operator/1, Block RAM/2(wr_addr)
  Block RAM/1(rd_data) -> hps/1, Multiport Switch1/2
  AND/1 -> Delay2/1
  mode/1 -> Multiport Switch/1
  address/1 -> Relational Operator/2, Delay/1, Block RAM/4(rd_addr)
  edge/1 -> Delay1/1
  Multiport Switch/1 -> Block RAM/1(wr_data)
  Delay3/1 -> Multiport Switch1/3
  Multiport Switch1/1 -> Add/2
  Add/1 -> Multiport Switch/3, Delay3/1

== system gm_parallel_lht_vnl/Parallel LHT/Parallel LHT Accumulator/Accumulator with Switches/Accumulator_instance144 ==
  mode : Inport  OutDataTypeStr=boolean  PortDimensions=1  SampleTime=6.66666666666667e-09
  address : Inport  Port=2  OutDataTypeStr=fixdt(0, 9, 0)  PortDimensions=1  SampleTime=6.66666666666667e-09
  edge : Inport  Port=3  OutDataTypeStr=boolean  PortDimensions=1  SampleTime=6.66666666666667e-09
  AND : Logic  IconShape=distinctive  AllPortsSameDT=off  OutDataTypeStr=boolean
  Add : Sum  OutDataTypeStr=fixdt(0, ceil(log2(maxRho*2)), 0)
  Block RAM : Subsystem
  Delay{,1..3} (4 alike) : Delay  DelayLength=1
  Multiport Switch : MultiPortSwitch  DataPortOrder=Zero-based contiguous  Inputs=2  zeroidx=on
  Multiport Switch1 : MultiPortSwitch  DataPortOrder=Zero-based contiguous  Inputs=2  zeroidx=on
  Relational Operator : RelationalOperator  Operator===  OutDataTypeStr=boolean  RndMeth=Simplest
  Vote : Constant  OutDataTypeStr=fixdt(0,1,0)  SampleTime=-1
  Zero : Constant  OutDataTypeStr=fixdt(0,1,0)  SampleTime=-1
  hps : Outport
  wires:
  Zero/1 -> Multiport Switch/2
  Vote/1 -> Add/1
  Relational Operator/1 -> AND/2
  Delay2/1 -> Multiport Switch1/1
  Delay1/1 -> AND/1, Block RAM/3(wr_en)
  Delay/1 -> Relational Operator/1, Block RAM/2(wr_addr)
  Block RAM/1(rd_data) -> hps/1, Multiport Switch1/2
  AND/1 -> Delay2/1
  mode/1 -> Multiport Switch/1
  address/1 -> Relational Operator/2, Delay/1, Block RAM/4(rd_addr)
  edge/1 -> Delay1/1
  Multiport Switch/1 -> Block RAM/1(wr_data)
  Delay3/1 -> Multiport Switch1/3
  Multiport Switch1/1 -> Add/2
  Add/1 -> Multiport Switch/3, Delay3/1

== system gm_parallel_lht_vnl/Parallel LHT/Parallel LHT Accumulator/Accumulator with Switches/Accumulator_instance145 ==
  mode : Inport  OutDataTypeStr=boolean  PortDimensions=1  SampleTime=6.66666666666667e-09
  address : Inport  Port=2  OutDataTypeStr=fixdt(0, 9, 0)  PortDimensions=1  SampleTime=6.66666666666667e-09
  edge : Inport  Port=3  OutDataTypeStr=boolean  PortDimensions=1  SampleTime=6.66666666666667e-09
  AND : Logic  IconShape=distinctive  AllPortsSameDT=off  OutDataTypeStr=boolean
  Add : Sum  OutDataTypeStr=fixdt(0, ceil(log2(maxRho*2)), 0)
  Block RAM : Subsystem
  Delay{,1..3} (4 alike) : Delay  DelayLength=1
  Multiport Switch : MultiPortSwitch  DataPortOrder=Zero-based contiguous  Inputs=2  zeroidx=on
  Multiport Switch1 : MultiPortSwitch  DataPortOrder=Zero-based contiguous  Inputs=2  zeroidx=on
  Relational Operator : RelationalOperator  Operator===  OutDataTypeStr=boolean  RndMeth=Simplest
  Vote : Constant  OutDataTypeStr=fixdt(0,1,0)  SampleTime=-1
  Zero : Constant  OutDataTypeStr=fixdt(0,1,0)  SampleTime=-1
  hps : Outport
  wires:
  Zero/1 -> Multiport Switch/2
  Vote/1 -> Add/1
  Relational Operator/1 -> AND/2
  Delay2/1 -> Multiport Switch1/1
  Delay1/1 -> AND/1, Block RAM/3(wr_en)
  Delay/1 -> Relational Operator/1, Block RAM/2(wr_addr)
  Block RAM/1(rd_data) -> hps/1, Multiport Switch1/2
  AND/1 -> Delay2/1
  mode/1 -> Multiport Switch/1
  address/1 -> Relational Operator/2, Delay/1, Block RAM/4(rd_addr)
  edge/1 -> Delay1/1
  Multiport Switch/1 -> Block RAM/1(wr_data)
  Delay3/1 -> Multiport Switch1/3
  Multiport Switch1/1 -> Add/2
  Add/1 -> Multiport Switch/3, Delay3/1

== system gm_parallel_lht_vnl/Parallel LHT/Parallel LHT Accumulator/Accumulator with Switches/Accumulator_instance146 ==
  mode : Inport  OutDataTypeStr=boolean  PortDimensions=1  SampleTime=6.66666666666667e-09
  address : Inport  Port=2  OutDataTypeStr=fixdt(0, 9, 0)  PortDimensions=1  SampleTime=6.66666666666667e-09
  edge : Inport  Port=3  OutDataTypeStr=boolean  PortDimensions=1  SampleTime=6.66666666666667e-09
  AND : Logic  IconShape=distinctive  AllPortsSameDT=off  OutDataTypeStr=boolean
  Add : Sum  OutDataTypeStr=fixdt(0, ceil(log2(maxRho*2)), 0)
  Block RAM : Subsystem
  Delay{,1..3} (4 alike) : Delay  DelayLength=1
  Multiport Switch : MultiPortSwitch  DataPortOrder=Zero-based contiguous  Inputs=2  zeroidx=on
  Multiport Switch1 : MultiPortSwitch  DataPortOrder=Zero-based contiguous  Inputs=2  zeroidx=on
  Relational Operator : RelationalOperator  Operator===  OutDataTypeStr=boolean  RndMeth=Simplest
  Vote : Constant  OutDataTypeStr=fixdt(0,1,0)  SampleTime=-1
  Zero : Constant  OutDataTypeStr=fixdt(0,1,0)  SampleTime=-1
  hps : Outport
  wires:
  Zero/1 -> Multiport Switch/2
  Vote/1 -> Add/1
  Relational Operator/1 -> AND/2
  Delay2/1 -> Multiport Switch1/1
  Delay1/1 -> AND/1, Block RAM/3(wr_en)
  Delay/1 -> Relational Operator/1, Block RAM/2(wr_addr)
  Block RAM/1(rd_data) -> hps/1, Multiport Switch1/2
  AND/1 -> Delay2/1
  mode/1 -> Multiport Switch/1
  address/1 -> Relational Operator/2, Delay/1, Block RAM/4(rd_addr)
  edge/1 -> Delay1/1
  Multiport Switch/1 -> Block RAM/1(wr_data)
  Delay3/1 -> Multiport Switch1/3
  Multiport Switch1/1 -> Add/2
  Add/1 -> Multiport Switch/3, Delay3/1

== system gm_parallel_lht_vnl/Parallel LHT/Parallel LHT Accumulator/Accumulator with Switches/Accumulator_instance147 ==
  mode : Inport  OutDataTypeStr=boolean  PortDimensions=1  SampleTime=6.66666666666667e-09
  address : Inport  Port=2  OutDataTypeStr=fixdt(0, 9, 0)  PortDimensions=1  SampleTime=6.66666666666667e-09
  edge : Inport  Port=3  OutDataTypeStr=boolean  PortDimensions=1  SampleTime=6.66666666666667e-09
  AND : Logic  IconShape=distinctive  AllPortsSameDT=off  OutDataTypeStr=boolean
  Add : Sum  OutDataTypeStr=fixdt(0, ceil(log2(maxRho*2)), 0)
  Block RAM : Subsystem
  Delay{,1..3} (4 alike) : Delay  DelayLength=1
  Multiport Switch : MultiPortSwitch  DataPortOrder=Zero-based contiguous  Inputs=2  zeroidx=on
  Multiport Switch1 : MultiPortSwitch  DataPortOrder=Zero-based contiguous  Inputs=2  zeroidx=on
  Relational Operator : RelationalOperator  Operator===  OutDataTypeStr=boolean  RndMeth=Simplest
  Vote : Constant  OutDataTypeStr=fixdt(0,1,0)  SampleTime=-1
  Zero : Constant  OutDataTypeStr=fixdt(0,1,0)  SampleTime=-1
  hps : Outport
  wires:
  Zero/1 -> Multiport Switch/2
  Vote/1 -> Add/1
  Relational Operator/1 -> AND/2
  Delay2/1 -> Multiport Switch1/1
  Delay1/1 -> AND/1, Block RAM/3(wr_en)
  Delay/1 -> Relational Operator/1, Block RAM/2(wr_addr)
  Block RAM/1(rd_data) -> hps/1, Multiport Switch1/2
  AND/1 -> Delay2/1
  mode/1 -> Multiport Switch/1
  address/1 -> Relational Operator/2, Delay/1, Block RAM/4(rd_addr)
  edge/1 -> Delay1/1
  Multiport Switch/1 -> Block RAM/1(wr_data)
  Delay3/1 -> Multiport Switch1/3
  Multiport Switch1/1 -> Add/2
  Add/1 -> Multiport Switch/3, Delay3/1

== system gm_parallel_lht_vnl/Parallel LHT/Parallel LHT Accumulator/Accumulator with Switches/Accumulator_instance148 ==
  mode : Inport  OutDataTypeStr=boolean  PortDimensions=1  SampleTime=6.66666666666667e-09
  address : Inport  Port=2  OutDataTypeStr=fixdt(0, 9, 0)  PortDimensions=1  SampleTime=6.66666666666667e-09
  edge : Inport  Port=3  OutDataTypeStr=boolean  PortDimensions=1  SampleTime=6.66666666666667e-09
  AND : Logic  IconShape=distinctive  AllPortsSameDT=off  OutDataTypeStr=boolean
  Add : Sum  OutDataTypeStr=fixdt(0, ceil(log2(maxRho*2)), 0)
  Block RAM : Subsystem
  Delay{,1..3} (4 alike) : Delay  DelayLength=1
  Multiport Switch : MultiPortSwitch  DataPortOrder=Zero-based contiguous  Inputs=2  zeroidx=on
  Multiport Switch1 : MultiPortSwitch  DataPortOrder=Zero-based contiguous  Inputs=2  zeroidx=on
  Relational Operator : RelationalOperator  Operator===  OutDataTypeStr=boolean  RndMeth=Simplest
  Vote : Constant  OutDataTypeStr=fixdt(0,1,0)  SampleTime=-1
  Zero : Constant  OutDataTypeStr=fixdt(0,1,0)  SampleTime=-1
  hps : Outport
  wires:
  Zero/1 -> Multiport Switch/2
  Vote/1 -> Add/1
  Relational Operator/1 -> AND/2
  Delay2/1 -> Multiport Switch1/1
  Delay1/1 -> AND/1, Block RAM/3(wr_en)
  Delay/1 -> Relational Operator/1, Block RAM/2(wr_addr)
  Block RAM/1(rd_data) -> hps/1, Multiport Switch1/2
  AND/1 -> Delay2/1
  mode/1 -> Multiport Switch/1
  address/1 -> Relational Operator/2, Delay/1, Block RAM/4(rd_addr)
  edge/1 -> Delay1/1
  Multiport Switch/1 -> Block RAM/1(wr_data)
  Delay3/1 -> Multiport Switch1/3
  Multiport Switch1/1 -> Add/2
  Add/1 -> Multiport Switch/3, Delay3/1

== system gm_parallel_lht_vnl/Parallel LHT/Parallel LHT Accumulator/Accumulator with Switches/Accumulator_instance149 ==
  mode : Inport  OutDataTypeStr=boolean  PortDimensions=1  SampleTime=6.66666666666667e-09
  address : Inport  Port=2  OutDataTypeStr=fixdt(0, 9, 0)  PortDimensions=1  SampleTime=6.66666666666667e-09
  edge : Inport  Port=3  OutDataTypeStr=boolean  PortDimensions=1  SampleTime=6.66666666666667e-09
  AND : Logic  IconShape=distinctive  AllPortsSameDT=off  OutDataTypeStr=boolean
  Add : Sum  OutDataTypeStr=fixdt(0, ceil(log2(maxRho*2)), 0)
  Block RAM : Subsystem
  Delay{,1..3} (4 alike) : Delay  DelayLength=1
  Multiport Switch : MultiPortSwitch  DataPortOrder=Zero-based contiguous  Inputs=2  zeroidx=on
  Multiport Switch1 : MultiPortSwitch  DataPortOrder=Zero-based contiguous  Inputs=2  zeroidx=on
  Relational Operator : RelationalOperator  Operator===  OutDataTypeStr=boolean  RndMeth=Simplest
  Vote : Constant  OutDataTypeStr=fixdt(0,1,0)  SampleTime=-1
  Zero : Constant  OutDataTypeStr=fixdt(0,1,0)  SampleTime=-1
  hps : Outport
  wires:
  Zero/1 -> Multiport Switch/2
  Vote/1 -> Add/1
  Relational Operator/1 -> AND/2
  Delay2/1 -> Multiport Switch1/1
  Delay1/1 -> AND/1, Block RAM/3(wr_en)
  Delay/1 -> Relational Operator/1, Block RAM/2(wr_addr)
  Block RAM/1(rd_data) -> hps/1, Multiport Switch1/2
  AND/1 -> Delay2/1
  mode/1 -> Multiport Switch/1
  address/1 -> Relational Operator/2, Delay/1, Block RAM/4(rd_addr)
  edge/1 -> Delay1/1
  Multiport Switch/1 -> Block RAM/1(wr_data)
  Delay3/1 -> Multiport Switch1/3
  Multiport Switch1/1 -> Add/2
  Add/1 -> Multiport Switch/3, Delay3/1

== system gm_parallel_lht_vnl/Parallel LHT/Parallel LHT Accumulator/Accumulator with Switches/Accumulator_instance15 ==
  mode : Inport  OutDataTypeStr=boolean  PortDimensions=1  SampleTime=6.66666666666667e-09
  address : Inport  Port=2  OutDataTypeStr=fixdt(0, 9, 0)  PortDimensions=1  SampleTime=6.66666666666667e-09
  edge : Inport  Port=3  OutDataTypeStr=boolean  PortDimensions=1  SampleTime=6.66666666666667e-09
  AND : Logic  IconShape=distinctive  AllPortsSameDT=off  OutDataTypeStr=boolean
  Add : Sum  OutDataTypeStr=fixdt(0, ceil(log2(maxRho*2)), 0)
  Block RAM : Subsystem
  Delay{,1..3} (4 alike) : Delay  DelayLength=1
  Multiport Switch : MultiPortSwitch  DataPortOrder=Zero-based contiguous  Inputs=2  zeroidx=on
  Multiport Switch1 : MultiPortSwitch  DataPortOrder=Zero-based contiguous  Inputs=2  zeroidx=on
  Relational Operator : RelationalOperator  Operator===  OutDataTypeStr=boolean  RndMeth=Simplest
  Vote : Constant  OutDataTypeStr=fixdt(0,1,0)  SampleTime=-1
  Zero : Constant  OutDataTypeStr=fixdt(0,1,0)  SampleTime=-1
  hps : Outport
  wires:
  Zero/1 -> Multiport Switch/2
  Vote/1 -> Add/1
  Relational Operator/1 -> AND/2
  Delay2/1 -> Multiport Switch1/1
  Delay1/1 -> AND/1, Block RAM/3(wr_en)
  Delay/1 -> Relational Operator/1, Block RAM/2(wr_addr)
  Block RAM/1(rd_data) -> hps/1, Multiport Switch1/2
  AND/1 -> Delay2/1
  mode/1 -> Multiport Switch/1
  address/1 -> Relational Operator/2, Delay/1, Block RAM/4(rd_addr)
  edge/1 -> Delay1/1
  Multiport Switch/1 -> Block RAM/1(wr_data)
  Delay3/1 -> Multiport Switch1/3
  Multiport Switch1/1 -> Add/2
  Add/1 -> Multiport Switch/3, Delay3/1

== system gm_parallel_lht_vnl/Parallel LHT/Parallel LHT Accumulator/Accumulator with Switches/Accumulator_instance150 ==
  mode : Inport  OutDataTypeStr=boolean  PortDimensions=1  SampleTime=6.66666666666667e-09
  address : Inport  Port=2  OutDataTypeStr=fixdt(0, 9, 0)  PortDimensions=1  SampleTime=6.66666666666667e-09
  edge : Inport  Port=3  OutDataTypeStr=boolean  PortDimensions=1  SampleTime=6.66666666666667e-09
  AND : Logic  IconShape=distinctive  AllPortsSameDT=off  OutDataTypeStr=boolean
  Add : Sum  OutDataTypeStr=fixdt(0, ceil(log2(maxRho*2)), 0)
  Block RAM : Subsystem
  Delay{,1..3} (4 alike) : Delay  DelayLength=1
  Multiport Switch : MultiPortSwitch  DataPortOrder=Zero-based contiguous  Inputs=2  zeroidx=on
  Multiport Switch1 : MultiPortSwitch  DataPortOrder=Zero-based contiguous  Inputs=2  zeroidx=on
  Relational Operator : RelationalOperator  Operator===  OutDataTypeStr=boolean  RndMeth=Simplest
  Vote : Constant  OutDataTypeStr=fixdt(0,1,0)  SampleTime=-1
  Zero : Constant  OutDataTypeStr=fixdt(0,1,0)  SampleTime=-1
  hps : Outport
  wires:
  Zero/1 -> Multiport Switch/2
  Vote/1 -> Add/1
  Relational Operator/1 -> AND/2
  Delay2/1 -> Multiport Switch1/1
  Delay1/1 -> AND/1, Block RAM/3(wr_en)
  Delay/1 -> Relational Operator/1, Block RAM/2(wr_addr)
  Block RAM/1(rd_data) -> hps/1, Multiport Switch1/2
  AND/1 -> Delay2/1
  mode/1 -> Multiport Switch/1
  address/1 -> Relational Operator/2, Delay/1, Block RAM/4(rd_addr)
  edge/1 -> Delay1/1
  Multiport Switch/1 -> Block RAM/1(wr_data)
  Delay3/1 -> Multiport Switch1/3
  Multiport Switch1/1 -> Add/2
  Add/1 -> Multiport Switch/3, Delay3/1

== system gm_parallel_lht_vnl/Parallel LHT/Parallel LHT Accumulator/Accumulator with Switches/Accumulator_instance151 ==
  mode : Inport  OutDataTypeStr=boolean  PortDimensions=1  SampleTime=6.66666666666667e-09
  address : Inport  Port=2  OutDataTypeStr=fixdt(0, 9, 0)  PortDimensions=1  SampleTime=6.66666666666667e-09
  edge : Inport  Port=3  OutDataTypeStr=boolean  PortDimensions=1  SampleTime=6.66666666666667e-09
  AND : Logic  IconShape=distinctive  AllPortsSameDT=off  OutDataTypeStr=boolean
  Add : Sum  OutDataTypeStr=fixdt(0, ceil(log2(maxRho*2)), 0)
  Block RAM : Subsystem
  Delay{,1..3} (4 alike) : Delay  DelayLength=1
  Multiport Switch : MultiPortSwitch  DataPortOrder=Zero-based contiguous  Inputs=2  zeroidx=on
  Multiport Switch1 : MultiPortSwitch  DataPortOrder=Zero-based contiguous  Inputs=2  zeroidx=on
  Relational Operator : RelationalOperator  Operator===  OutDataTypeStr=boolean  RndMeth=Simplest
  Vote : Constant  OutDataTypeStr=fixdt(0,1,0)  SampleTime=-1
  Zero : Constant  OutDataTypeStr=fixdt(0,1,0)  SampleTime=-1
  hps : Outport
  wires:
  Zero/1 -> Multiport Switch/2
  Vote/1 -> Add/1
  Relational Operator/1 -> AND/2
  Delay2/1 -> Multiport Switch1/1
  Delay1/1 -> AND/1, Block RAM/3(wr_en)
  Delay/1 -> Relational Operator/1, Block RAM/2(wr_addr)
  Block RAM/1(rd_data) -> hps/1, Multiport Switch1/2
  AND/1 -> Delay2/1
  mode/1 -> Multiport Switch/1
  address/1 -> Relational Operator/2, Delay/1, Block RAM/4(rd_addr)
  edge/1 -> Delay1/1
  Multiport Switch/1 -> Block RAM/1(wr_data)
  Delay3/1 -> Multiport Switch1/3
  Multiport Switch1/1 -> Add/2
  Add/1 -> Multiport Switch/3, Delay3/1
